simulink model "CDCJournalModel"  (R2017a)
settings: Solver=VariableStepAuto  StartTime=0.0  StopTime=10.0  RelTol=1e-3
PreLoadFcn:
  | preLoadCallback
StartFcn:
  | startCallback
StopFcn:
  | tsc=dataset2TSC(logsout);
undefined symbols (not defined in the file or in its folder): aeroTable, p
libraries: library x7, vrlib x1
settings Model: Creator=M.Cobb  LastModifiedBy=M.Cobb
settings DataIOCC: SaveFormat=Structure

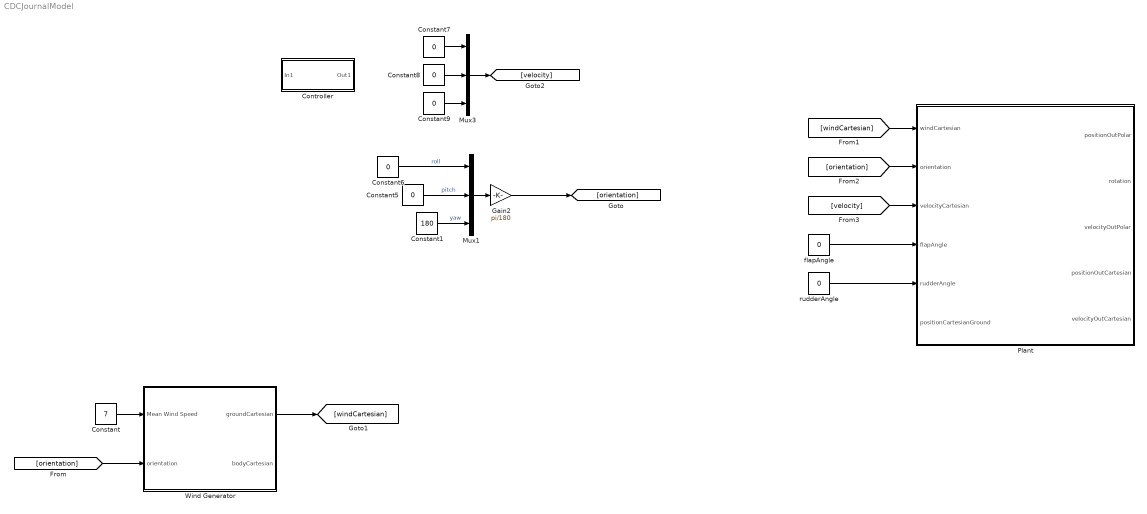
== system CDCJournalModel ==
  Constant : Constant  Value=7
  Constant1 : Constant  Value=180
  Constant{5..9} (5 alike) : Constant  Value=0
  Controller : Subsystem
  Gain2 : Gain  Gain=pi/180
  Mux1 : Mux  Inputs=3
  Mux3 : Mux  Inputs=3
  Plant : Subsystem
  Wind Generator : Subsystem
  flapAngle : Constant  Value=0
  rudderAngle : Constant  Value=0
  wires:
  Constant/1 -> Wind Generator/1(Mean Wind Speed)
  [orientation] -> Wind Generator/2(orientation)
  Constant5/1 -> Mux1/2  "pitch"
  Constant6/1 -> Mux1/1  "roll"
  Mux1/1 -> Gain2/1
  Constant1/1 -> Mux1/3  "yaw"
  Gain2/1 -> [orientation]
  Constant9/1 -> Mux3/3
  Constant8/1 -> Mux3/2
  Constant7/1 -> Mux3/1
  Wind Generator/1(groundCartesian) -> [windCartesian]
  [windCartesian] -> Plant/1(windCartesian)
  flapAngle/1 -> Plant/4(flapAngle)
  [orientation] -> Plant/2(orientation)
  Mux3/1 -> [velocity]
  [velocity] -> Plant/3(velocityCartesian)
  rudderAngle/1 -> Plant/5(rudderAngle)

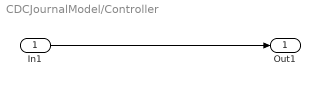
== system CDCJournalModel/Controller ==
  In1 : Inport
  Out1 : Outport
  wires:
  In1/1 -> Out1/1

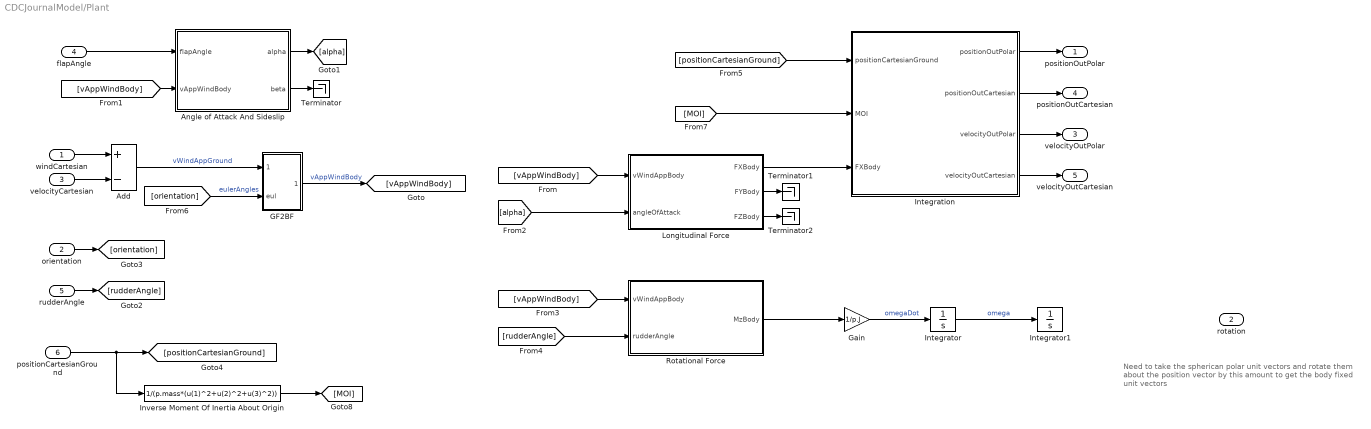
== system CDCJournalModel/Plant ==
  note: Need to take the spherican polar unit vectors and rotate
      | them about the position vector by this amount to get the body
      | fixed unit vectors
  windCartesian : Inport
  orientation : Inport  Port=2
  velocityCartesian : Inport  Port=3
  flapAngle : Inport  Port=4
  rudderAngle : Inport  Port=5
  positionCartesianGround : Inport  Port=6
  Add : Sum  Inputs=+-
  Angle of Attack And Sideslip : Subsystem
  GF2BF : Subsystem
  Gain : Gain  Gain=1/p.J
  Integration : Subsystem
  Integrator : Integrator
  Integrator1 : Integrator
  Inverse Moment Of Inertia About Origin : Fcn  Expr=1/(p.mass*(u(1)^2+u(2)^2+u(3)^2))
  Longitudinal Force : Subsystem
  Rotational Force : Subsystem
  Terminator : Terminator
  Terminator1 : Terminator
  Terminator2 : Terminator
  positionOutPolar : Outport
  rotation : Outport  Port=2
  velocityOutPolar : Outport  Port=3
  positionOutCartesian : Outport  Port=4
  velocityOutCartesian : Outport  Port=5
  wires:
  windCartesian/1 -> Add/1
  velocityCartesian/1 -> Add/2
  orientation/1 -> [orientation]
  flapAngle/1 -> Angle of Attack And Sideslip/1(flapAngle)
  [vAppWindBody] -> Angle of Attack And Sideslip/2(vAppWindBody)
  Angle of Attack And Sideslip/1(alpha) -> [alpha]
  Angle of Attack And Sideslip/2(beta) -> Terminator/1
  [vAppWindBody] -> Longitudinal Force/1(vWindAppBody)
  [alpha] -> Longitudinal Force/2(angleOfAttack)
  Add/1 -> GF2BF/1(vecIn)  "vWindAppGround"
  [orientation] -> GF2BF/2(eul)  "eulerAngles"
  GF2BF/1(vecOut) -> [vAppWindBody]  "vAppWindBody"
  [vAppWindBody] -> Rotational Force/1(vWindAppBody)
  rudderAngle/1 -> [rudderAngle]
  [rudderAngle] -> Rotational Force/2(rudderAngle)
  Rotational Force/1(MzBody) -> Gain/1
  Gain/1 -> Integrator/1  "omegaDot"
  Integrator/1 -> Integrator1/1  "omega"
  positionCartesianGround/1 -> Inverse Moment Of Inertia About Origin/1, [positionCartesianGround]
  Inverse Moment Of Inertia About Origin/1 -> [MOI]
  Longitudinal Force/2(FYBody) -> Terminator1/1
  Longitudinal Force/3(FZBody) -> Terminator2/1
  Integration/1(positionOutPolar) -> positionOutPolar/1
  [positionCartesianGround] -> Integration/1("positionCartesianGround ")
  Integration/2(positionOutCartesian) -> positionOutCartesian/1
  Integration/3(velocityOutPolar) -> velocityOutPolar/1
  Integration/4(velocityOutCartesian) -> velocityOutCartesian/1
  Longitudinal Force/1(FXBody) -> Integration/3(FXBody)
  [MOI] -> Integration/2(MOI)

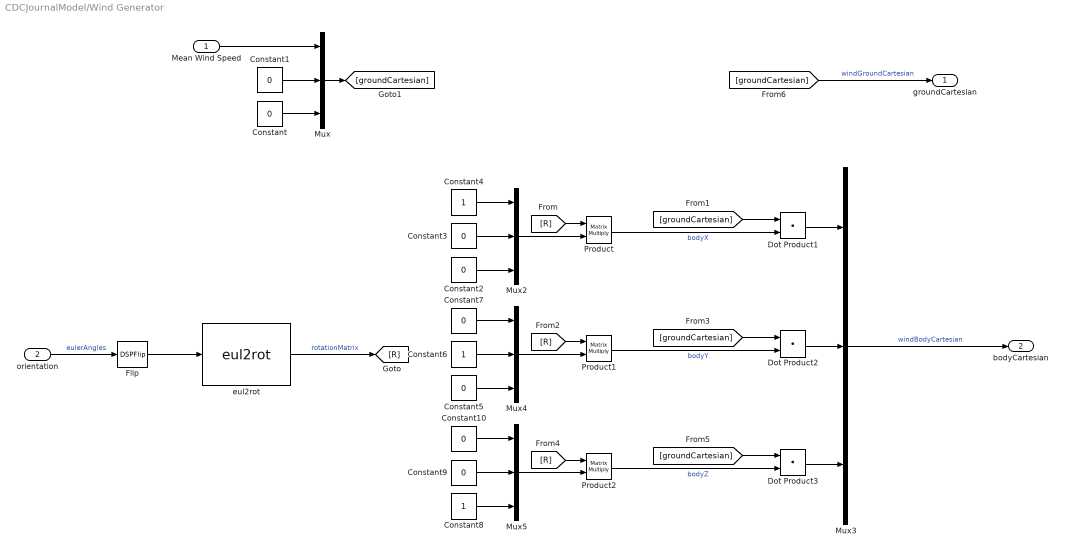
== system CDCJournalModel/Wind Generator ==
  Mean Wind Speed : Inport  Unit=m/s
  orientation : Inport  Port=2  Unit=rad
  Constant{,1..3,5,7,9..10} (8 alike) : Constant  Value=0
  Constant4 : Constant
  Constant6 : Constant
  Constant8 : Constant
  Dot Product1 : DotProduct  InputSameDT=on  OutDataTypeStr=Inherit: Inherit via internal rule
  Dot Product2 : DotProduct  InputSameDT=on  OutDataTypeStr=Inherit: Inherit via internal rule
  Dot Product3 : DotProduct  InputSameDT=on  OutDataTypeStr=Inherit: Inherit via internal rule
  Flip : DSPFlip
  Mux{,2..5} (5 alike) : Mux  Inputs=3
  Product : Product  Multiplication=Matrix(*)
  Product1 : Product  Multiplication=Matrix(*)
  Product2 : Product  Multiplication=Matrix(*)
  eul2rot : library/eul2rot
  groundCartesian : Outport
  bodyCartesian : Outport  Port=2
  wires:
  Mean Wind Speed/1 -> Mux/1
  Constant1/1 -> Mux/2
  Constant/1 -> Mux/3
  orientation/1 -> Flip/1  "eulerAngles"
  Constant2/1 -> Mux2/3
  Constant3/1 -> Mux2/2
  Constant4/1 -> Mux2/1
  Mux2/1 -> Product/2
  eul2rot/1 -> [R]  "rotationMatrix"
  [R] -> Product/1
  Product/1 -> Dot Product1/2  "bodyX"
  Mux/1 -> [groundCartesian]
  [groundCartesian] -> Dot Product1/1
  Dot Product1/1 -> Mux3/1
  Mux3/1 -> bodyCartesian/1  "windBodyCartesian"
  Constant6/1 -> Mux4/2
  Mux4/1 -> Product1/2
  Constant5/1 -> Mux4/3
  Product1/1 -> Dot Product2/2  "bodyY"
  [R] -> Product1/1
  [groundCartesian] -> Dot Product2/1
  Constant7/1 -> Mux4/1
  [groundCartesian] -> Dot Product3/1
  [R] -> Product2/1
  Constant9/1 -> Mux5/2
  Constant8/1 -> Mux5/3
  Mux5/1 -> Product2/2
  Product2/1 -> Dot Product3/2  "bodyZ"
  Dot Product2/1 -> Mux3/2
  Dot Product3/1 -> Mux3/3
  Constant10/1 -> Mux5/1
  [groundCartesian] -> groundCartesian/1  "windGroundCartesian"
  Flip/1 -> eul2rot/1

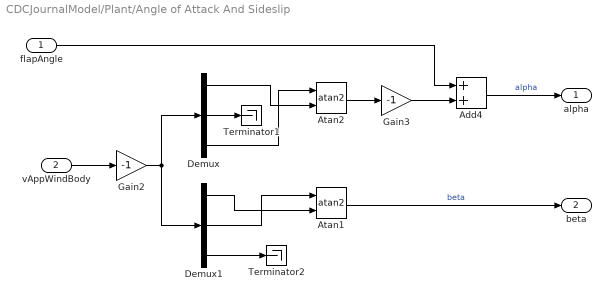
== system CDCJournalModel/Plant/Angle of Attack And Sideslip ==
  flapAngle : Inport
  vAppWindBody : Inport  Port=2
  Add4 : Sum
  Atan1 : Trigonometry  Operator=atan2
  Atan2 : Trigonometry  Operator=atan2
  Demux : Demux  Outputs=3
  Demux1 : Demux  Outputs=3
  Gain2 : Gain  Gain=-1
  Gain3 : Gain  Gain=-1
  Terminator1 : Terminator
  Terminator2 : Terminator
  alpha : Outport
  beta : Outport  Port=2
  wires:
  Gain3/1 -> Add4/2
  vAppWindBody/1 -> Gain2/1
  Demux/1 -> Atan2/2
  Atan2/1 -> Gain3/1
  Atan1/1 -> beta/1  "beta"
  Demux/3 -> Atan2/1
  Add4/1 -> alpha/1  "alpha"
  Demux/2 -> Terminator1/1
  flapAngle/1 -> Add4/1
  Demux1/2 -> Atan1/1
  Demux1/1 -> Atan1/2
  Demux1/3 -> Terminator2/1
  Gain2/1 -> Demux1/1, Demux/1

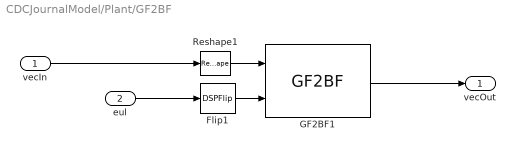
== system CDCJournalModel/Plant/GF2BF ==
  vecIn : Inport
  eul : Inport  Port=2
  Flip1 : DSPFlip
  GF2BF1 : library/GF2BF
  Reshape1 : Reshape  OutputDimensions=[3 1]
  vecOut : Outport
  wires:
  Reshape1/1 -> GF2BF1/1
  GF2BF1/1 -> vecOut/1
  Flip1/1 -> GF2BF1/2
  eul/1 -> Flip1/1
  vecIn/1 -> Reshape1/1

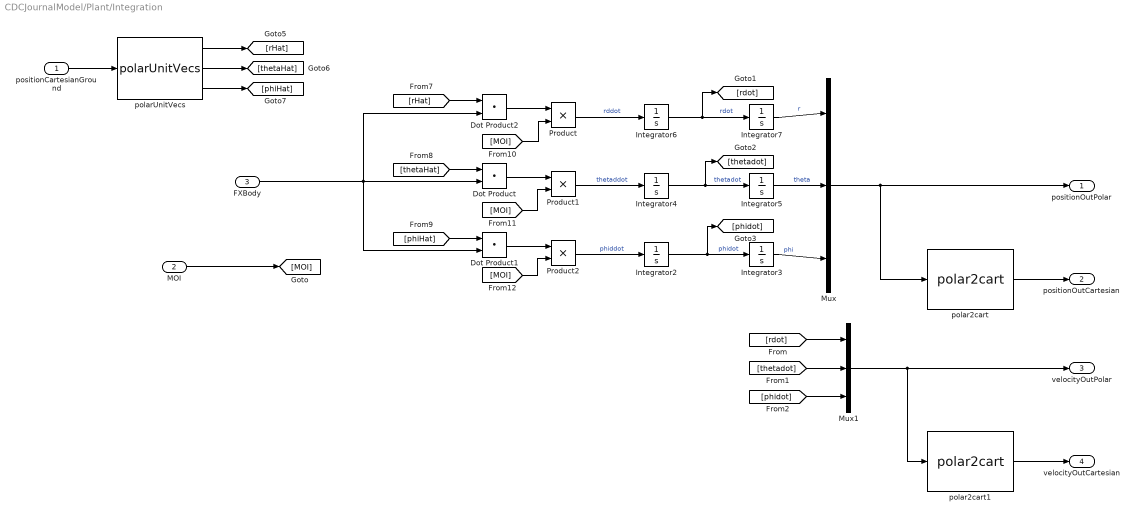
== system CDCJournalModel/Plant/Integration ==
  "positionCartesianGround " : Inport
  MOI : Inport  Port=2
  FXBody : Inport  Port=3
  Dot Product : DotProduct  InputSameDT=on  OutDataTypeStr=Inherit: Inherit via internal rule
  Dot Product1 : DotProduct  InputSameDT=on  OutDataTypeStr=Inherit: Inherit via internal rule
  Dot Product2 : DotProduct  InputSameDT=on  OutDataTypeStr=Inherit: Inherit via internal rule
  Integrator{2..7} (6 alike) : Integrator
  Mux : Mux  Inputs=3
  Mux1 : Mux  Inputs=3
  Product : Product
  Product1 : Product
  Product2 : Product
  polar2cart : library/polar2cart
  polar2cart1 : library/polar2cart
  polarUnitVecs : library/polarUnitVecs
  positionOutPolar : Outport
  positionOutCartesian : Outport  Port=2
  velocityOutPolar : Outport  Port=3
  velocityOutCartesian : Outport  Port=4
  wires:
  polarUnitVecs/3 -> [phiHat]
  FXBody/1 -> Dot Product2/2, Dot Product1/2, Dot Product/2
  [MOI] -> Product1/2
  Product/1 -> Integrator6/1  "rddot"
  Integrator6/1 -> [rdot], Integrator7/1  "rdot"
  Integrator2/1 -> [phidot], Integrator3/1  "phidot"
  Dot Product1/1 -> Product2/1
  Product2/1 -> Integrator2/1  "phiddot"
  Product1/1 -> Integrator4/1  "thetaddot"
  Integrator5/1 -> Mux/2  "theta"
  [MOI] -> Product/2
  Integrator4/1 -> [thetadot], Integrator5/1  "thetadot"
  [rHat] -> Dot Product2/1
  [thetaHat] -> Dot Product/1
  Integrator7/1 -> Mux/1  "r"
  polarUnitVecs/1 -> [rHat]
  Dot Product2/1 -> Product/1
  "positionCartesianGround "/1 -> polarUnitVecs/1
  [MOI] -> Product2/2
  [phiHat] -> Dot Product1/1
  Integrator3/1 -> Mux/3  "phi"
  Dot Product/1 -> Product1/1
  polarUnitVecs/2 -> [thetaHat]
  polar2cart/1 -> positionOutCartesian/1
  polar2cart1/1 -> velocityOutCartesian/1
  Mux/1 -> polar2cart/1, positionOutPolar/1
  Mux1/1 -> polar2cart1/1, velocityOutPolar/1
  [rdot] -> Mux1/1
  [thetadot] -> Mux1/2
  [phidot] -> Mux1/3
  MOI/1 -> [MOI]

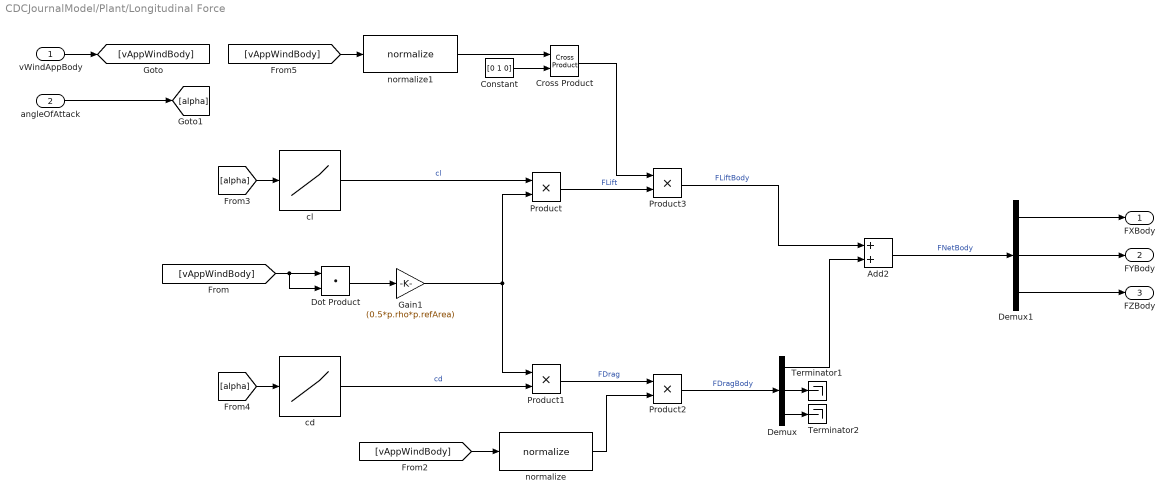
== system CDCJournalModel/Plant/Longitudinal Force ==
  vWindAppBody : Inport
  angleOfAttack : Inport  Port=2
  Add2 : Sum
  Constant : Constant  Value=[0 1 0]
  Cross Product : vrlib/Utilities/Cross Product
      settings: SourceProductBaseCode=VR
  Demux : Demux  Outputs=3
  Demux1 : Demux  Outputs=3
  Dot Product : DotProduct  InputSameDT=on  OutDataTypeStr=Inherit: Inherit via internal rule
  Gain1 : Gain  Gain=(0.5*p.rho*p.refArea)
  Product{,1..3} (4 alike) : Product
  Terminator1 : Terminator
  Terminator2 : Terminator
  cd : Lookup_n-D  NumberOfTableDimensions=1  BreakpointsForDimension1=aeroTable.alpha  Table=aeroTable.cd  InternalRulePriority=Speed  RndMeth=Simplest  InputSameDT=on
  cl : Lookup_n-D  NumberOfTableDimensions=1  BreakpointsForDimension1=aeroTable.alpha  Table=aeroTable.cl  InternalRulePriority=Speed  RndMeth=Simplest  InputSameDT=on
  normalize : library/normalize
  normalize1 : library/normalize
  FXBody : Outport
  FYBody : Outport  Port=2
  FZBody : Outport  Port=3
  wires:
  Product1/1 -> Product2/1  "FDrag"
  normalize/1 -> Product2/2
  [vAppWindBody] -> normalize1/1
  Demux/3 -> Terminator2/1
  Product2/1 -> Demux/1  "FDragBody"
  [vAppWindBody] -> normalize/1
  Product/1 -> Product3/2  "FLift"
  Cross Product/1 -> Product3/1
  Constant/1 -> Cross Product/2
  Product3/1 -> Add2/1  "FLiftBody"
  normalize1/1 -> Cross Product/1
  [alpha] -> cd/1
  Dot Product/1 -> Gain1/1
  [alpha] -> cl/1
  cl/1 -> Product/1  "cl"
  [vAppWindBody] -> Dot Product/2, Dot Product/1
  Demux/2 -> Terminator1/1
  Gain1/1 -> Product/2, Product1/1
  cd/1 -> Product1/2  "cd"
  vWindAppBody/1 -> [vAppWindBody]
  angleOfAttack/1 -> [alpha]
  Add2/1 -> Demux1/1  "FNetBody"
  Demux/1 -> Add2/2
  Demux1/1 -> FXBody/1
  Demux1/2 -> FYBody/1
  Demux1/3 -> FZBody/1

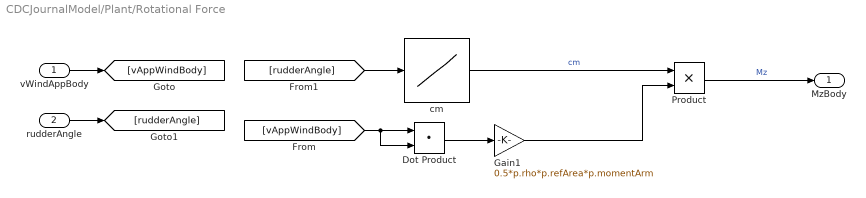
== system CDCJournalModel/Plant/Rotational Force ==
  vWindAppBody : Inport
  rudderAngle : Inport  Port=2
  Dot Product : DotProduct  InputSameDT=on  OutDataTypeStr=Inherit: Inherit via internal rule
  Gain1 : Gain  Gain=0.5*p.rho*p.refArea*p.momentArm
  Product : Product
  cm : Lookup_n-D  NumberOfTableDimensions=1  BreakpointsForDimension1=aeroTable.rudderAngle  Table=aeroTable.cm  InternalRulePriority=Speed  RndMeth=Simplest  InputSameDT=on
  MzBody : Outport
  wires:
  Dot Product/1 -> Gain1/1
  [rudderAngle] -> cm/1
  cm/1 -> Product/1  "cm"
  [vAppWindBody] -> Dot Product/2, Dot Product/1
  Gain1/1 -> Product/2
  vWindAppBody/1 -> [vAppWindBody]
  rudderAngle/1 -> [rudderAngle]
  Product/1 -> MzBody/1  "Mz"
